simulink model "wind_draiden_final"  (R2020a)
settings: Solver=VariableStepAuto  StartTime=0.0  StopTime=10.0  RelTol=1e-3
undefined symbols (not defined in the file or in its folder): ln, MAV
libraries: simulink x6
settings Model: Creator=Tamer  LastModifiedBy=ZelDen
settings SolverCC: ZeroCrossControl=DisableAll
settings DataIOCC: SaveOutput=off  SaveTime=off
settings GRTTargetCC: CombineOutputUpdateFcns=off  MatFileLogging=off

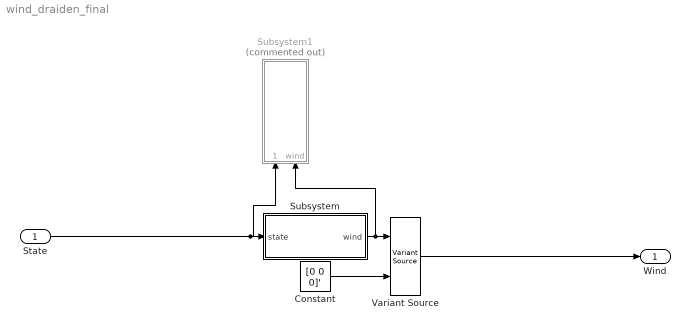
== system wind_draiden_final ==
  State : Inport  PortDimensions=[12; 1]
  Constant : Constant  Value=[0 0 0]'
  Subsystem : Subsystem
  Subsystem1 : Subsystem  Commented=on
  Variant Source : VariantSource
  Wind : Outport
  wires:
  Variant Source/1 -> Wind/1
  State/1 -> Subsystem1/1(state), Subsystem/1(state)
  Constant/1 -> Variant Source/2
  Subsystem/1(wind) -> Variant Source/1, Subsystem1/2(wind)

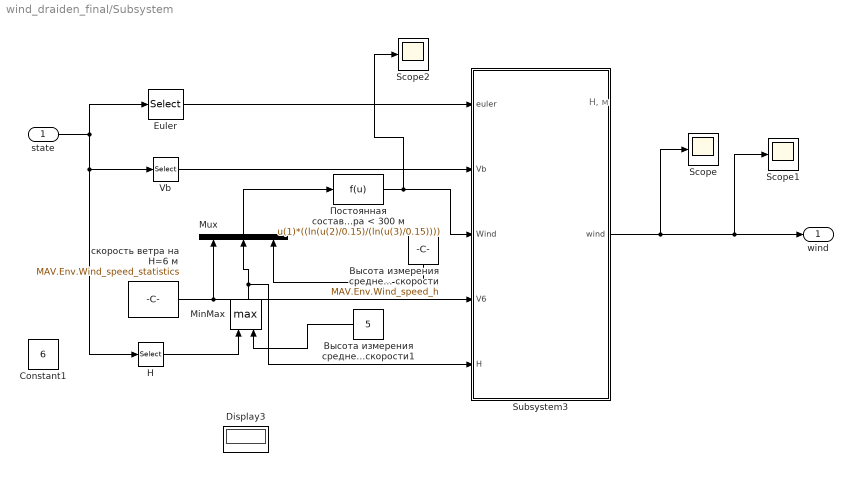
== system wind_draiden_final/Subsystem ==
  note: Н, м
  state : Inport
  "    Постоянная составляющая скорости ветра < 300 м" : Fcn  Expr=u(1)*((ln(u(2)/0.15)/(ln(u(3)/0.15))))
  Constant1 : Constant  Value=6
  Display3 : Display
  Euler : Selector  InputPortWidth=12  IndexOptions=Index vector (dialog)  Indices=[7, 8, 9]  OutputSizes=1
  H : Selector  InputPortWidth=12  IndexOptions=Index vector (dialog)  Indices=[2]  OutputSizes=1
  MinMax : MinMax  Function=max  Inputs=2
  Mux : Mux  Inputs=3
  Scope : Scope
  Scope1 : Scope
  Scope2 : Scope
  Subsystem3 : Subsystem
  Vb : Selector  InputPortWidth=12  IndexOptions=Index vector (dialog)  Indices=[4 5 6]  OutputSizes=1
  Высота измерения среднегодовой скорости : Constant  Value=MAV.Env.Wind_speed_h
  Высота измерения среднегодовой скорости1 : Constant  Value=5
  "скорость ветра на Н=6 м " : Constant  Value=MAV.Env.Wind_speed_statistics
  wind : Outport
  wires:
  Высота измерения среднегодовой скорости/1 -> Mux/3
  Mux/1 -> "    Постоянная составляющая скорости ветра < 300 м"/1
  "    Постоянная составляющая скорости ветра < 300 м"/1 -> Scope2/1, Subsystem3/3(Wind)
  "скорость ветра на Н=6 м "/1 -> Mux/1, Subsystem3/4(V6)
  Vb/1 -> Subsystem3/2(Vb)
  Euler/1 -> Subsystem3/1(euler)
  state/1 -> H/1, Vb/1, Euler/1
  Subsystem3/1(wind) -> Scope/1, Scope1/1, wind/1
  MinMax/1 -> Subsystem3/5(H), Mux/2
  Высота измерения среднегодовой скорости1/1 -> MinMax/2
  H/1 -> MinMax/1

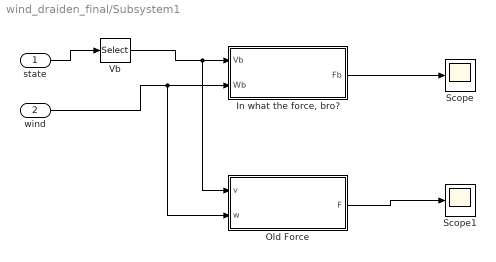
== system wind_draiden_final/Subsystem1 ==
  state : Inport
  wind : Inport  Port=2
  "In what the force, bro?" : MATLAB Function  TreatAsAtomicUnit=on
  Old Force : MATLAB Function  TreatAsAtomicUnit=on
  Scope : Scope
  Scope1 : Scope
  Vb : Selector  InputPortWidth=12  IndexOptions=Index vector (dialog)  Indices=[4:6]  OutputSizes=1
  wires:
  state/1 -> Vb/1
  Vb/1 -> Old Force/1(v), "In what the force, bro?"/1(Vb)
  wind/1 -> Old Force/2(w), "In what the force, bro?"/2(Wb)
  "In what the force, bro?"/1(Fb) -> Scope/1
  Old Force/1(F) -> Scope1/1

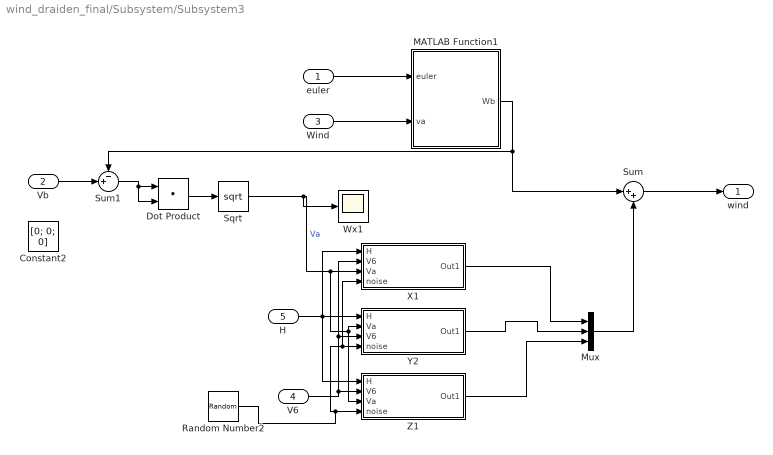
== system wind_draiden_final/Subsystem/Subsystem3 ==
  euler : Inport
  Vb : Inport  Port=2
  Wind : Inport  Port=3
  V6 : Inport  Port=4
  H : Inport  Port=5
  Constant2 : Constant  Value=[0; 0; 0]
  Dot Product : DotProduct  InputSameDT=on  OutDataTypeStr=Inherit: Inherit via internal rule
  MATLAB Function1 : MATLAB Function  TreatAsAtomicUnit=on
  Mux : Mux  Inputs=3
  Random Number2 : RandomNumber  SampleTime=0.1
  Sqrt : Sqrt  SaturateOnIntegerOverflow=on
  Sum : Sum  Inputs=|++
  Sum1 : Sum  Inputs=-+|
  Wx1 : Scope
  X1 : Subsystem  TreatAsAtomicUnit=on
  Y2 : Subsystem  TreatAsAtomicUnit=on
  Z1 : Subsystem  TreatAsAtomicUnit=on
  wind : Outport
  wires:
  euler/1 -> MATLAB Function1/1(euler)
  Wind/1 -> MATLAB Function1/2(va)
  MATLAB Function1/1(Wb) -> Sum/1, Sum1/1
  Mux/1 -> Sum/2
  Sum/1 -> wind/1
  Sqrt/1 -> Wx1/1, Y2/2(Va), Z1/3(Va), X1/3(Va)  "Va"
  H/1 -> Y2/1(H), X1/1(H), Z1/1(H)
  V6/1 -> X1/2(V6), Y2/3(V6), Z1/2(V6)
  Z1/1(Out1) -> Mux/3
  X1/1(Out1) -> Mux/1
  Y2/1(Out1) -> Mux/2
  Random Number2/1 -> Y2/4(noise), X1/4(noise), Z1/4(noise)
  Sum1/1 -> Dot Product/1, Dot Product/2
  Dot Product/1 -> Sqrt/1
  Vb/1 -> Sum1/2

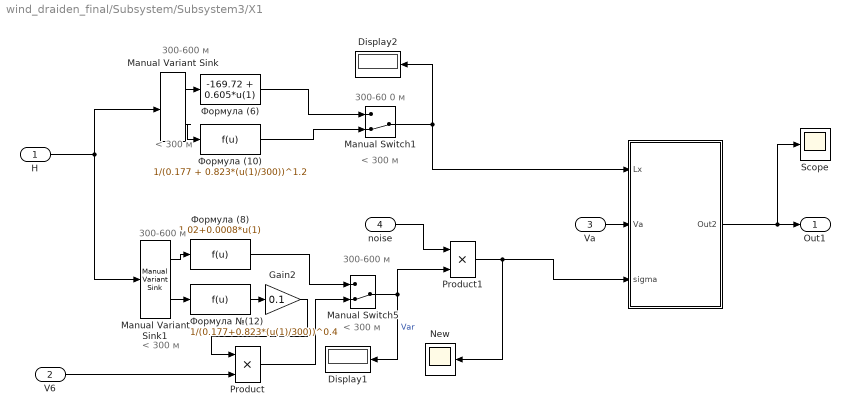
== system wind_draiden_final/Subsystem/Subsystem3/X1 ==
  note: < 300 м
  note: 300-600 м
  note: < 300 м
  note: < 300 м
  note: 300-600 м
  note: < 300 м
  note: 300-60 0 м
  note: 300-600 м
  H : Inport
  V6 : Inport  Port=2
  Va : Inport  Port=3
  noise : Inport  Port=4
  " " : Subsystem
  Display1 : Display
  Display2 : Display
  Gain2 : Gain  Gain=0.1
  Manual Variant Sink : simulink/Signal Routing/Manual Variant Sink  NumChoices=2  LabelModeActiveChoice=V_2
  Manual Variant Sink1 : simulink/Signal Routing/Manual Variant Sink  NumChoices=2  LabelModeActiveChoice=V_2
  Manual Switch1 : ManualSwitch  CurrentSetting=0
  Manual Switch5 : ManualSwitch  CurrentSetting=0
  New : Scope
  Product : Product
  Product1 : Product
  Scope : Scope
  Формула (10) : Fcn  Expr=1/(0.177 + 0.823*(u(1)/300))^1.2
  Формула (6) : Fcn  Expr=-169.72 + 0.605*u(1)
  Формула (8) : Fcn  Expr=1.02+0.0008*u(1)
  Формула №(12) : Fcn  Expr=1/(0.177+0.823*(u(1)/300))^0.4
  Out1 : Outport
  wires:
  Формула №(12)/1 -> Gain2/1
  Формула (8)/1 -> Manual Switch5/1
  Manual Variant Sink/2 -> Формула (10)/1
  Manual Variant Sink1/1 -> Формула (8)/1
  Gain2/1 -> Product/1
  Manual Variant Sink1/2 -> Формула №(12)/1
  Manual Switch5/1 -> Display1/1, Product1/2  "Var"
  " "/1(Out2) -> Scope/1, Out1/1
  Product/1 -> Manual Switch5/2
  Формула (6)/1 -> Manual Switch1/1
  H/1 -> Manual Variant Sink1/1, Manual Variant Sink/1
  V6/1 -> Product/2
  Manual Variant Sink/1 -> Формула (6)/1
  Manual Switch1/1 -> " "/1(Lx), Display2/1
  Формула (10)/1 -> Manual Switch1/2
  Va/1 -> " "/2(Va)
  Product1/1 -> New/1, " "/3("sigma ")
  noise/1 -> Product1/1

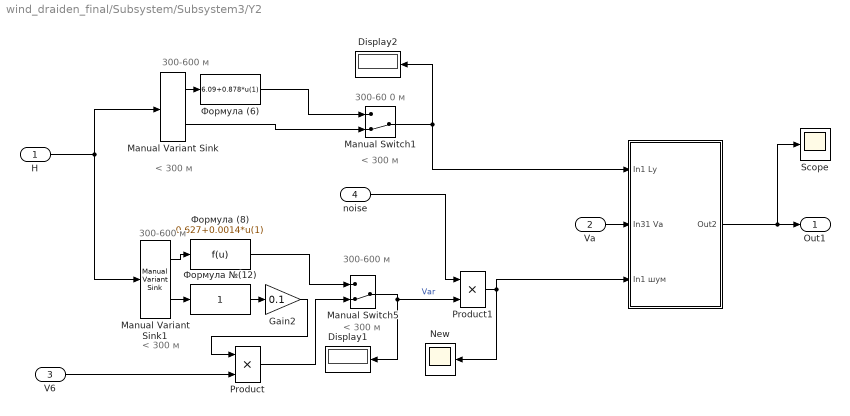
== system wind_draiden_final/Subsystem/Subsystem3/Y2 ==
  note: < 300 м
  note: 300-600 м
  note: < 300 м
  note: < 300 м
  note: 300-600 м
  note: < 300 м
  note: 300-60 0 м
  note: 300-600 м
  H : Inport
  Va : Inport  Port=2
  V6 : Inport  Port=3
  noise : Inport  Port=4
  " " : Subsystem
  Display1 : Display
  Display2 : Display
  Gain2 : Gain  Gain=0.1
  Manual Variant Sink : simulink/Signal Routing/Manual Variant Sink  NumChoices=2  LabelModeActiveChoice=V_2
  Manual Variant Sink1 : simulink/Signal Routing/Manual Variant Sink  NumChoices=2  LabelModeActiveChoice=V_2
  Manual Switch1 : ManualSwitch  CurrentSetting=0
  Manual Switch5 : ManualSwitch  CurrentSetting=0
  New : Scope
  Product : Product
  Product1 : Product
  Scope : Scope
  Формула (6) : Fcn  Expr=6.09+0.878*u(1)
  Формула (8) : Fcn  Expr=0.627+0.0014*u(1)
  Формула №(12) : Fcn  Expr=1
  Out1 : Outport
  wires:
  noise/1 -> Product1/1
  Формула №(12)/1 -> Gain2/1
  Формула (8)/1 -> Manual Switch5/1
  Product1/1 -> New/1, " "/3("In1 шум ")
  Manual Variant Sink1/1 -> Формула (8)/1
  Gain2/1 -> Product/1
  Manual Variant Sink1/2 -> Формула №(12)/1
  Manual Switch5/1 -> Product1/2, Display1/1  "Var"
  " "/1(Out2) -> Scope/1, Out1/1
  Product/1 -> Manual Switch5/2
  Формула (6)/1 -> Manual Switch1/1
  H/1 -> Manual Variant Sink1/1, Manual Variant Sink/1
  V6/1 -> Product/2
  Manual Variant Sink/1 -> Формула (6)/1
  Manual Switch1/1 -> " "/1(In1 Ly), Display2/1
  Manual Variant Sink/2 -> Manual Switch1/2
  Va/1 -> " "/2(In31 Va)

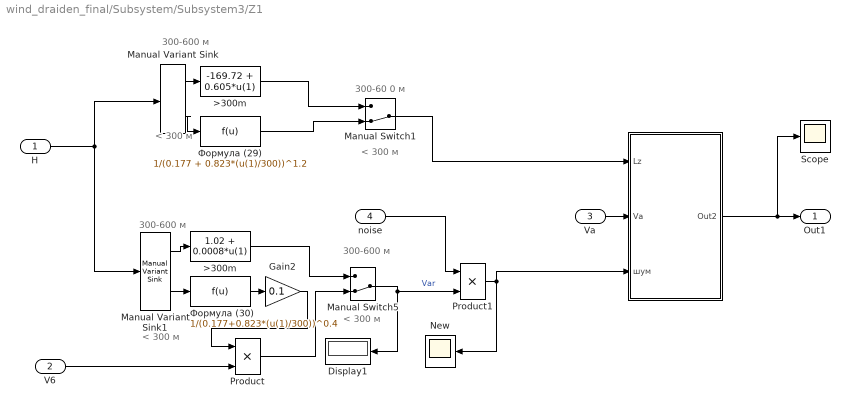
== system wind_draiden_final/Subsystem/Subsystem3/Z1 ==
  note: < 300 м
  note: 300-600 м
  note: < 300 м
  note: < 300 м
  note: 300-600 м
  note: < 300 м
  note: 300-60 0 м
  note: 300-600 м
  H : Inport
  V6 : Inport  Port=2
  Va : Inport  Port=3
  noise : Inport  Port=4
  " " : Subsystem
  " >300m" : Fcn  Expr=-169.72 + 0.605*u(1)
  >300m : Fcn  Expr=1.02 + 0.0008*u(1)
  Display1 : Display
  Gain2 : Gain  Gain=0.1
  Manual Variant Sink : simulink/Signal Routing/Manual Variant Sink  NumChoices=2  LabelModeActiveChoice=V_2
  Manual Variant Sink1 : simulink/Signal Routing/Manual Variant Sink  NumChoices=2  LabelModeActiveChoice=V_2
  Manual Switch1 : ManualSwitch  CurrentSetting=0
  Manual Switch5 : ManualSwitch  CurrentSetting=0
  New : Scope
  Product : Product
  Product1 : Product
  Scope : Scope
  Формула (29) : Fcn  Expr=1/(0.177 + 0.823*(u(1)/300))^1.2
  Формула (30) : Fcn  Expr=1/(0.177+0.823*(u(1)/300))^0.4
  Out1 : Outport
  wires:
  noise/1 -> Product1/1
  Формула (30)/1 -> Gain2/1
  >300m/1 -> Manual Switch5/1
  Product1/1 -> New/1, " "/3("шум ")
  Manual Variant Sink/2 -> Формула (29)/1
  Manual Variant Sink1/1 -> >300m/1
  Gain2/1 -> Product/1
  Manual Variant Sink1/2 -> Формула (30)/1
  Manual Switch5/1 -> Product1/2, Display1/1  "Var"
  " "/1(Out2) -> Scope/1, Out1/1
  Product/1 -> Manual Switch5/2
  " >300m"/1 -> Manual Switch1/1
  H/1 -> Manual Variant Sink1/1, Manual Variant Sink/1
  V6/1 -> Product/2
  Manual Variant Sink/1 -> " >300m"/1
  Manual Switch1/1 -> " "/1(Lz)
  Формула (29)/1 -> Manual Switch1/2
  Va/1 -> " "/2(Va)

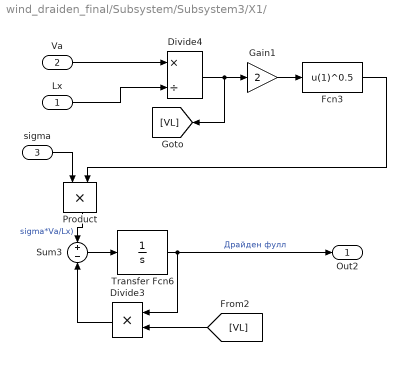
== system wind_draiden_final/Subsystem/Subsystem3/X1/  ==
  Lx : Inport
  Va : Inport  Port=2
  "sigma " : Inport  Port=3
  Divide3 : Product  Inputs=**
  Divide4 : Product  Inputs=*/
  Fcn3 : Fcn  Expr=u(1)^0.5
  Gain1 : Gain  Gain=2
  Product : Product
  Sum3 : Sum  Inputs=+-
  Transfer Fcn6 : TransferFcn  Denominator="[1  0]"
  Out2 : Outport
  wires:
  Divide4/1 -> [VL], Gain1/1
  Gain1/1 -> Fcn3/1
  Va/1 -> Divide4/1
  Lx/1 -> Divide4/2
  Transfer Fcn6/1 -> Out2/1, Divide3/1  "Драйден фулл"
  Divide3/1 -> Sum3/2
  Sum3/1 -> Transfer Fcn6/1
  [VL] -> Divide3/2
  Product/1 -> Sum3/1  "sigma*Va/Lx)"
  "sigma "/1 -> Product/1
  Fcn3/1 -> Product/2

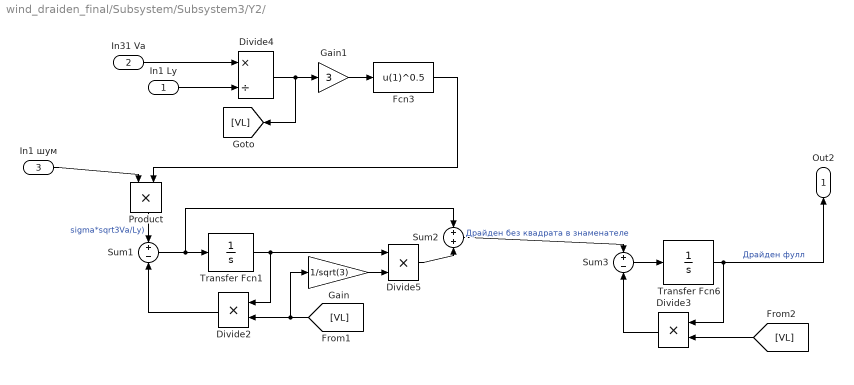
== system wind_draiden_final/Subsystem/Subsystem3/Y2/  ==
  In1 Ly : Inport
  In31 Va : Inport  Port=2
  "In1 шум " : Inport  Port=3
  Divide2 : Product  Inputs=**
  Divide3 : Product  Inputs=**
  Divide4 : Product  Inputs=*/
  Divide5 : Product  Inputs=**
  Fcn3 : Fcn  Expr=u(1)^0.5
  Gain : Gain  Gain=1/sqrt(3)
  Gain1 : Gain  Gain=3
  Product : Product
  Sum1 : Sum  Inputs=+-
  Sum2 : Sum
  Sum3 : Sum  Inputs=+-
  Transfer Fcn1 : TransferFcn  Denominator="[1  0]"
  Transfer Fcn6 : TransferFcn  Denominator="[1  0]"
  Out2 : Outport
  wires:
  Divide4/1 -> [VL], Gain1/1
  Sum1/1 -> Transfer Fcn1/1, Sum2/1
  Sum2/1 -> Sum3/1  "Драйден без квадрата в знаменателе"
  Transfer Fcn1/1 -> Divide2/1, Divide5/1
  Divide2/1 -> Sum1/2
  Gain1/1 -> Fcn3/1
  In31 Va/1 -> Divide4/1
  In1 Ly/1 -> Divide4/2
  [VL] -> Gain/1, Divide2/2
  Gain/1 -> Divide5/2
  Divide5/1 -> Sum2/2
  Transfer Fcn6/1 -> Out2/1, Divide3/1  "Драйден фулл"
  Divide3/1 -> Sum3/2
  Sum3/1 -> Transfer Fcn6/1
  [VL] -> Divide3/2
  "In1 шум "/1 -> Product/1
  Fcn3/1 -> Product/2
  Product/1 -> Sum1/1  "sigma*sqrt3Va/Ly)"

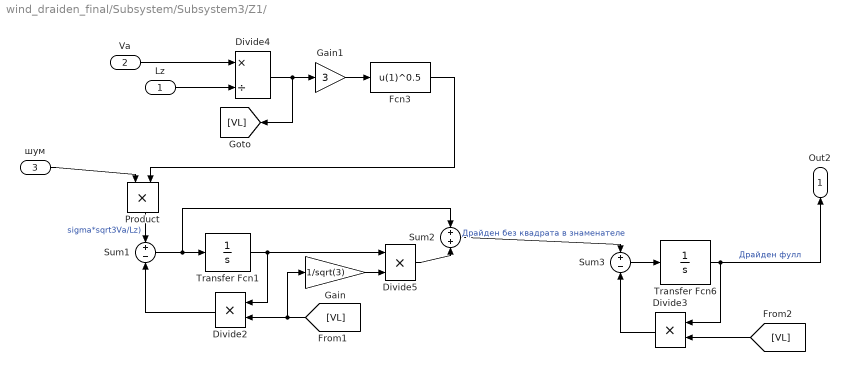
== system wind_draiden_final/Subsystem/Subsystem3/Z1/  ==
  Lz : Inport
  Va : Inport  Port=2
  "шум " : Inport  Port=3
  Divide2 : Product  Inputs=**
  Divide3 : Product  Inputs=**
  Divide4 : Product  Inputs=*/
  Divide5 : Product  Inputs=**
  Fcn3 : Fcn  Expr=u(1)^0.5
  Gain : Gain  Gain=1/sqrt(3)
  Gain1 : Gain  Gain=3
  Product : Product
  Sum1 : Sum  Inputs=+-
  Sum2 : Sum
  Sum3 : Sum  Inputs=+-
  Transfer Fcn1 : TransferFcn  Denominator="[1  0]"
  Transfer Fcn6 : TransferFcn  Denominator="[1  0]"
  Out2 : Outport
  wires:
  Divide4/1 -> [VL], Gain1/1
  Sum1/1 -> Transfer Fcn1/1, Sum2/1
  Sum2/1 -> Sum3/1  "Драйден без квадрата в знаменателе"
  Transfer Fcn1/1 -> Divide2/1, Divide5/1
  Divide2/1 -> Sum1/2
  Gain1/1 -> Fcn3/1
  Va/1 -> Divide4/1
  Lz/1 -> Divide4/2
  [VL] -> Gain/1, Divide2/2
  Gain/1 -> Divide5/2
  Divide5/1 -> Sum2/2
  Transfer Fcn6/1 -> Out2/1, Divide3/1  "Драйден фулл"
  Divide3/1 -> Sum3/2
  Sum3/1 -> Transfer Fcn6/1
  [VL] -> Divide3/2
  "шум "/1 -> Product/1
  Fcn3/1 -> Product/2
  Product/1 -> Sum1/1  "sigma*sqrt3Va/Lz)"

== matlab function wind_draiden_final/Subsystem1/In what the force, bro? ==
  data: Vb input; Fb output; Wb input
function Fb = AerialDrag(Vb, Wb)
    rho = 1.19;
    Va_vec = Vb - Wb;  % w - wind, v - ground speed; body frame
    Va = norm(Va_vec);
    alpha = atan2(Va_vec(2), Va_vec(1));    % attack angle
    beta = atan2(Va_vec(3), Va_vec(1));     % скольжения angle
    
    Va_0 = 10; % скорость, для которой рассчитаны зависимости сил
    rho_0 = 1.225;  % плотность воздуха при выведении зависимостей сил
%     C_0 = 0.715 / (0.5*rho_0*Va_0^2);  % if alpha = 0, beta = 0;
    % ----------------------------------------------------
    % alpha angle
    alpha = abs(alpha);
    alpha = sign(alpha)*mod(alpha, 180);
    alpha = alpha + 180 * sign(90-alpha)*(abs(alpha)>90);
    if alpha >= 0 && alpha <= 20
        F_xy = 0.6969 + 0.0022*(alpha+2.3409).^2;
    elseif alpha > 20 && alpha <= 90
        F_xy = -0.000435*alpha^2 + 0.098161*alpha - 0.007685;
%         C_d = 5.5300 - 4.3500e-04*(alpha - 112.8287)^2;
    elseif alpha >= -20 && alpha < 0
        F_xy = 0.6969 + 0.0022*(-alpha+2.3409).^2;
    else
        F_xy = 5.5300 - 4.3500e-04*(-alpha - 112.8287)^2;
    end
%     C_D_alpha = F_0 / (0.5*rho_0*Va_0^2) - C_0;
%     C_D_alpha = F_0 / (0.5*rho_0*Va_0^2);
        C_xy = F_xy / (0.5*rho_0*Va_0^2);
        C_x = C_xy * cos(alpha);
        C_y = C_xy * sin(alpha);
        
        
    
    %-----------------------------------------------------
    % beta angle
    b = abs(beta);
    b = sign(b)*mod(b, 180);
    b = b + 180 * sign(90-b)*(abs(b)>90);
    if b >= 0 && b <= 10
        F_xz = 2.81659e-7*b^6 - 5.42002e-6*b^5 + 0.0000194033*b^4 + 0.000149284*b^3 - 0.000766659*b^2 + 0.00100311*b + 0.715;
    elseif b > 10 && b <= 32
        F_xz = 0.000072941364*b^2+0.004725990899*b+0.676768850038;
    elseif b > 32 && b <= 47
        F_xz = 0.000014983590*b^3-0.002016505717*b^2+0.091338487517*b-0.446303186240;
    elseif b > 47 && b <= 66
        F_xz = -0.000005286789*b^3+0.000705178007*b^2-0.030877630605*b+1.390205322532;
    elseif b > 66 && b <= 90
        F_xz = 0.000000379469*b^3+0.000021666922*b^2-0.013615025702*b+1.599215019960;            
    else
        F_xz = 0;
    end
    C_xz = F_xz / (0.5*rho_0*Va_0^2);
    C_z = C_xz * sin(beta);
%     C_D_beta = F0 / (0.5*rho_0*Va_0^2) - C_0;
    
    
    % ----------------------------------------------
    % Drug force
%     F_D = 0.5*rho*Va^2 * (C_0 + alpha*C_D_alpha + beta*C_D_beta);
    
%     F_D = 0.5*rho*Va^2 * (C_D_alpha);
%     
%     Fa = [
%         (-1)*F_D;
%         0;
%         0;
%     ];  % в скоростной СК
%     c_a = cos(alpha); s_a = sin(alpha);
%     c_b = cos(beta); s_b = sin(beta);
%     % TODO: перепроверить, кто в кого переводитъ
%     R_a_b = [c_a*c_b -s_a*c_b s_b; s_a c_a 0; -c_a*s_b s_a*s_b c_b];    % из скоростной с связанную
% %     R_b_a = [ c_a s_a 0; -s_a c_a 0; 0 0 1];    % из связанной в скоростную
% %     Fb = R_b_a' * Fa;
%         Fb = R_a_b * Fa;
    Fb = (-1)*(1/2)*rho*Va^2 * [C_x; C_y; C_z];
end

== matlab function wind_draiden_final/Subsystem/Subsystem3/MATLAB Function1 ==
  data: euler input; Wb output; va input
function Wb = rotate_g_b(euler, va)
R = getRotationMatrix(euler);
% R = getRotationMatrix([0 0 0]);
vay=0; vaz=0;
Va = [-va; vay; vaz];
Wb = R*Va;

function R = getRotationMatrix(angles)
    phi = 1; t = 2; psi = 3; %indices
    s = sin(angles);
    c = cos(angles);
    R = [
        c(t)*c(psi) s(t)    -c(t)*s(psi);
        -c(phi)*s(t)*c(psi)+s(phi)*s(psi) c(phi)*c(t) c(phi)*s(t)*s(psi)+s(phi)*c(psi);
        s(phi)*s(t)*c(psi)+c(phi)*s(psi)  -s(phi)*c(t)    -s(psi)*s(t)*s(phi)+c(psi)*c(phi);
    ];

== matlab function wind_draiden_final/Subsystem1/Old Force ==
  data: v input; F output; w input
function F = AerialDrag(v, w)
    rho = 1.19;
    S = [5573 59852 6884] / (100*10)^2;
    C = 1.0;
    Va = v - w;  % w - wind, v - ground speed;
    % S - характерная площадь
    F = - C * rho * Va.^2/2 .* S';
end
